simulink model "x4DOF_Model"  (R2023a)
settings: Solver=VariableStepAuto  StartTime=0.0  StopTime=60  RelTol=1e-3
InitFcn:
  | data = readtable("car_rig_data.xlsx");
settings Model: Creator=Sebastian  LastModifiedBy=Sebastian

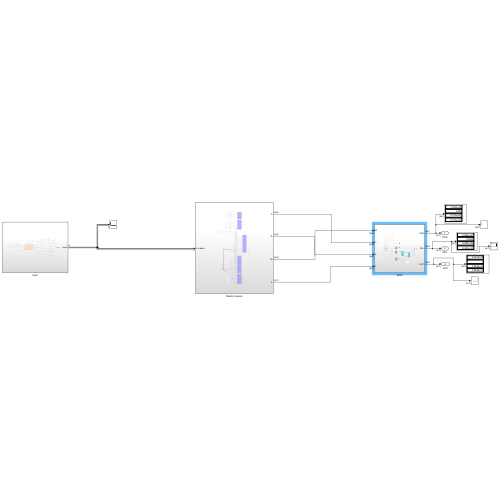
[thumbnail: Simulink's stored preview of the top-level diagram]
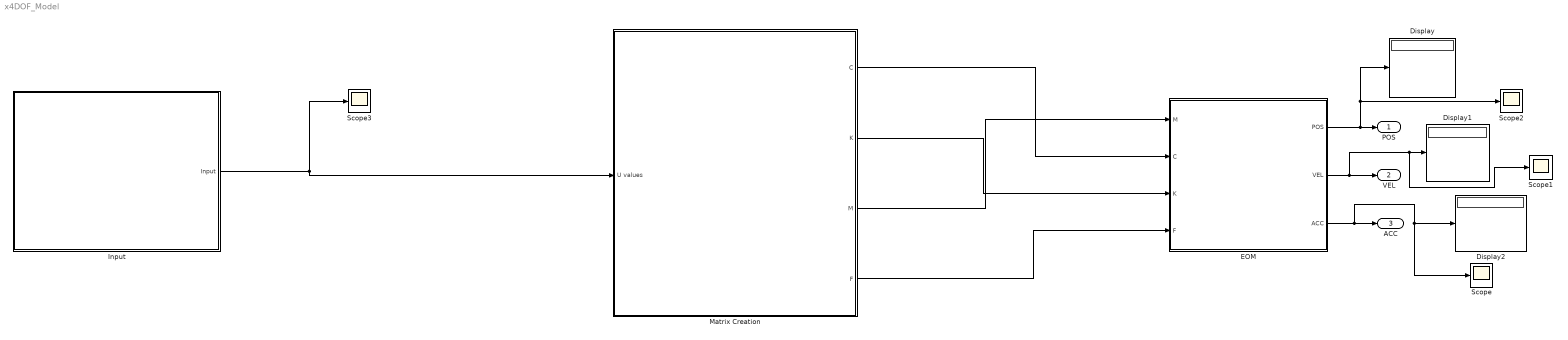
== system x4DOF_Model ==
  Display : Display
  Display1 : Display
  Display2 : Display
  EOM : Subsystem
  Input : Subsystem
  Matrix Creation : Subsystem
  Scope{,1..3} (4 alike) : Scope
  POS : Outport
  VEL : Outport  Port=2
  ACC : Outport  Port=3
  wires:
  Matrix Creation/3(M) -> EOM/1(M)
  Matrix Creation/2(K) -> EOM/3(K)
  Matrix Creation/1(C) -> EOM/2(C)
  Matrix Creation/4(F) -> EOM/4(F)
  EOM/1(POS) -> Scope2/1, Display/1, POS/1
  EOM/2(VEL) -> Scope1/1, Display1/1, VEL/1
  EOM/3(ACC) -> Scope/1, Display2/1, ACC/1
  Input/1(Input) -> Scope3/1, Matrix Creation/1(U values)

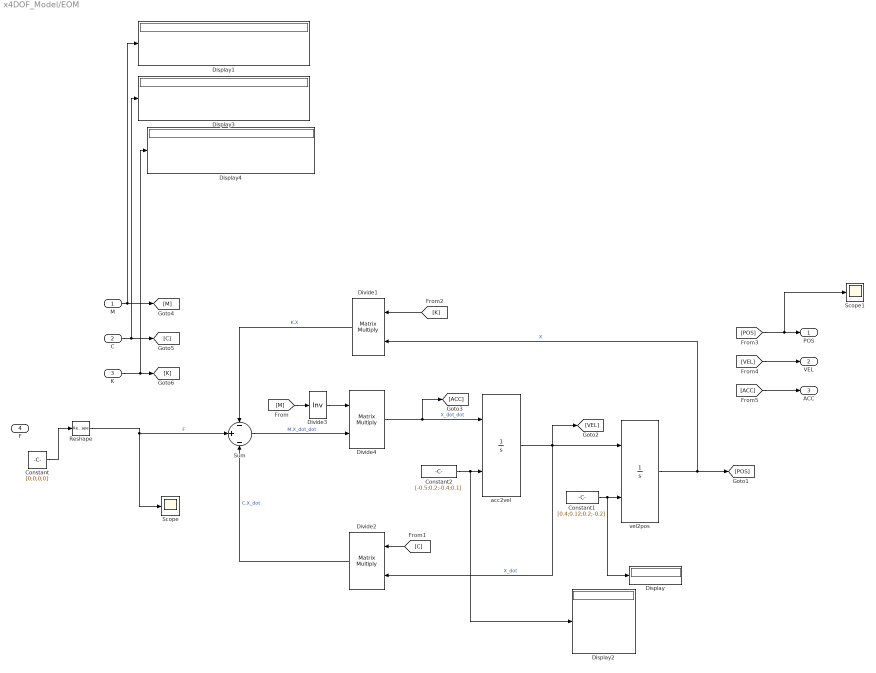
== system x4DOF_Model/EOM ==
  M : Inport
  C : Inport  Port=2
  K : Inport  Port=3
  F : Inport  Port=4
  Constant : Constant  Value=[0;0;0;0]
  Constant1 : Constant  Value=[0.4;0.12;0.2;-0.2]  VectorParams1D=off
  Constant2 : Constant  Value=[-0.5;0.2;-0.4;0.1]  VectorParams1D=off
  Display{,1..4} (5 alike) : Display
  Divide1 : Product  Multiplication=Matrix(*)
  Divide2 : Product  Multiplication=Matrix(*)
  Divide3 : Product  Inputs=/  Multiplication=Matrix(*)
  Divide4 : Product  Multiplication=Matrix(*)
  Reshape : Reshape  OutputDimensionality=Column vector (2-D)
  Scope : Scope
  Scope1 : Scope
  Sum : Sum  Inputs=-|+|-
  acc2vel : Integrator  InitialConditionSource=external
  vel2pos : Integrator  InitialConditionSource=external
  POS : Outport
  VEL : Outport  Port=2
  ACC : Outport  Port=3
  wires:
  Divide4/1 -> [ACC], acc2vel/1  "X_dot_dot"
  [C] -> Divide2/1
  vel2pos/1 -> [POS], Divide1/2  "X"
  Divide1/1 -> Sum/1  "K.X"
  acc2vel/1 -> vel2pos/1, [VEL], Divide2/2  "X_dot"
  [K] -> Divide1/1
  C/1 -> Display3/1, [C]
  Constant2/1 -> Display2/1, acc2vel/2
  [ACC] -> ACC/1
  [M] -> Divide3/1
  Constant1/1 -> Display/1, vel2pos/2
  [VEL] -> VEL/1
  Sum/1 -> Divide4/2  "M.X_dot_dot"
  Divide2/1 -> Sum/3  "C.X_dot"
  Divide3/1 -> Divide4/1
  Reshape/1 -> Scope/1, Sum/2  "F"
  [POS] -> Scope1/1, POS/1
  M/1 -> Display1/1, [M]
  K/1 -> Display4/1, [K]
  Constant/1 -> Reshape/1

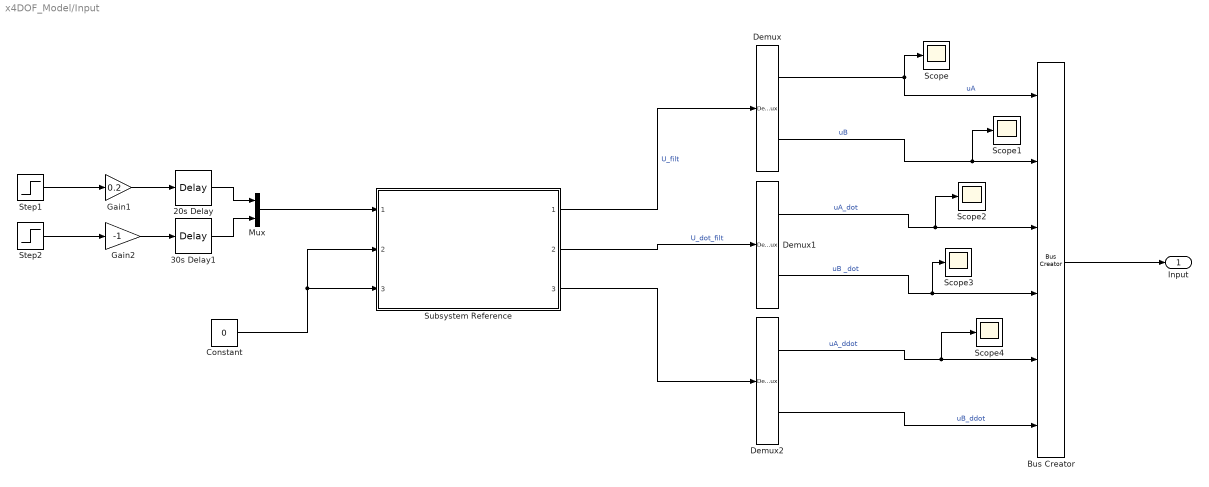
== system x4DOF_Model/Input ==
  20s Delay : TransportDelay  DelayTime=20
  30s Delay1 : TransportDelay  DelayTime=30
  Bus Creator : BusCreator  Inputs=6
  Constant : Constant  Value=0
  Demux : Demux  Outputs=2
  Demux1 : Demux  Outputs=2
  Demux2 : Demux  Outputs=2
  Gain1 : Gain  Gain=0.2
  Gain2 : Gain  Gain=-1
  Mux : Mux  Inputs=2
  Scope{,1..4} (5 alike) : Scope
  Step1 : Step  SampleTime=0
  Step2 : Step  SampleTime=0
  Subsystem Reference : Subsystem  ReferencedSubsystem=bh_COMPONENT_deriv_est  wn=2*pi*5000  p=1
  Input : Outport
  wires:
  Mux/1 -> Subsystem Reference/1
  Constant/1 -> Subsystem Reference/3, Subsystem Reference/2
  Subsystem Reference/1 -> Demux/1  "U_filt"
  Subsystem Reference/2 -> Demux1/1  "U_dot_filt"
  Subsystem Reference/3 -> Demux2/1
  Step2/1 -> Gain2/1
  Step1/1 -> Gain1/1
  Gain1/1 -> 20s Delay/1
  Gain2/1 -> 30s Delay1/1
  20s Delay/1 -> Mux/1
  30s Delay1/1 -> Mux/2
  Demux/1 -> Scope/1, Bus Creator/1  "uA"
  Demux/2 -> Bus Creator/2, Scope1/1  "uB"
  Demux1/1 -> Scope2/1, Bus Creator/3  "uA_dot"
  Demux1/2 -> Scope3/1, Bus Creator/4  "uB _dot"
  Demux2/1 -> Scope4/1, Bus Creator/5  "uA_ddot"
  Demux2/2 -> Bus Creator/6  "uB_ddot"
  Bus Creator/1 -> Input/1

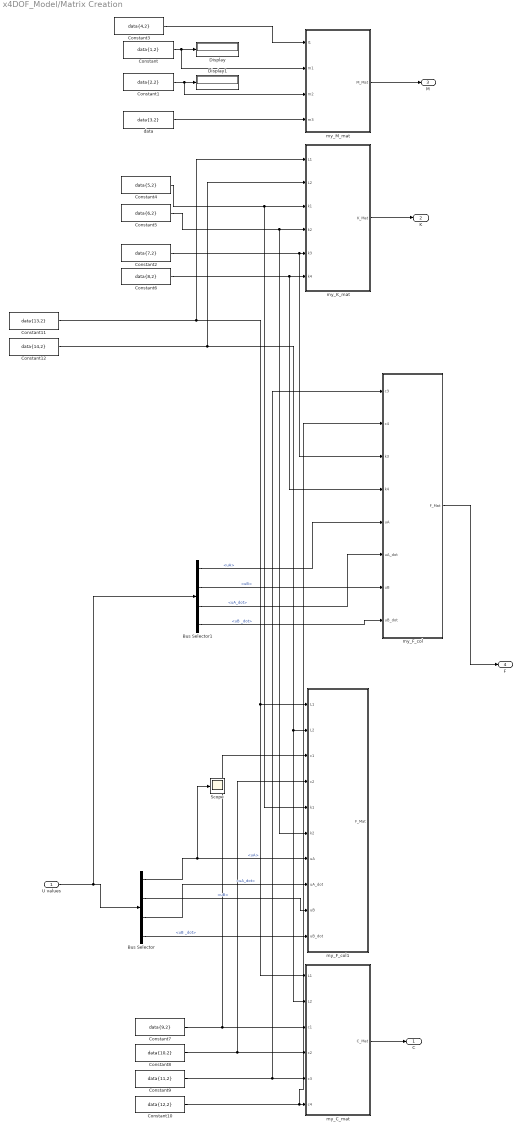
== system x4DOF_Model/Matrix Creation ==
  U values : Inport
  Bus Selector : BusSelector  OutputSignals=uA,uB,uA_dot,uB _dot
  Bus Selector1 : BusSelector  OutputSignals=uA,uB,uA_dot,uB _dot
  Constant : Constant  Value=data{1,2}
  Constant1 : Constant  Value=data{2,2}
  Constant10 : Constant  Value=data{12,2}
  Constant11 : Constant  Value=data{13,2}
  Constant12 : Constant  Value=data{14,2}
  Constant2 : Constant  Value=data{7,2}
  Constant3 : Constant  Value=data{4,2}
  Constant4 : Constant  Value=data{5,2}
  Constant5 : Constant  Value=data{6,2}
  Constant6 : Constant  Value=data{8,2}
  Constant7 : Constant  Value=data{9,2}
  Constant8 : Constant  Value=data{10,2}
  Constant9 : Constant  Value=data{11,2}
  Display : Display
  Display1 : Display
  Scope : Scope
  data : Constant  Value=data{3,2}
  my_C_mat : MATLAB Function  TreatAsAtomicUnit=on
  my_F_col : MATLAB Function  TreatAsAtomicUnit=on
  my_F_col1 : MATLAB Function  TreatAsAtomicUnit=on
  my_K_mat : MATLAB Function  TreatAsAtomicUnit=on
  my_M_mat : MATLAB Function  TreatAsAtomicUnit=on
  C : Outport
  K : Outport  Port=2
  M : Outport  Port=3
  F : Outport  Port=4
  wires:
  my_C_mat/1(C_Mat) -> C/1
  my_K_mat/1(K_Mat) -> K/1
  my_M_mat/1(M_Mat) -> M/1
  Constant/1 -> my_M_mat/2(m1), Display/1
  Constant1/1 -> my_M_mat/3(m2), Display1/1
  Constant3/1 -> my_M_mat/1(I1)
  data/1 -> my_M_mat/4(m3)
  Constant5/1 -> my_K_mat/4(k2), my_F_col1/6(k2)
  Constant4/1 -> my_F_col1/5(k1), my_K_mat/3(k1)
  Constant2/1 -> my_F_col/3(k3), my_K_mat/5(k3)
  Constant6/1 -> my_F_col/4(k4), my_K_mat/6(k4)
  Constant10/1 -> my_F_col/2(c4), my_C_mat/6(c4)
  Constant9/1 -> my_F_col/1(c3), my_C_mat/5(c3)
  Constant8/1 -> my_F_col1/4(c2), my_C_mat/4(c2)
  Constant7/1 -> my_C_mat/3(c1), my_F_col1/3(c1)
  Constant11/1 -> my_K_mat/1(L1), my_C_mat/1(L1), my_F_col1/1(L1)
  Constant12/1 -> my_K_mat/2(L2), my_C_mat/2(L2), my_F_col1/2(L2)
  Bus Selector/2 -> my_F_col1/9(uB)  "<uB>"
  U values/1 -> Bus Selector1/1, Bus Selector/1
  Bus Selector/4 -> my_F_col1/10(uB_dot)  "<uB _dot>"
  Bus Selector/3 -> my_F_col1/8(uA_dot)  "<uA_dot>"
  Bus Selector/1 -> Scope/1, my_F_col1/7(uA)  "<uA>"
  Bus Selector1/4 -> my_F_col/8(uB_dot)  "<uB _dot>"
  Bus Selector1/2 -> my_F_col/7(uB)  "<uB>"
  Bus Selector1/3 -> my_F_col/6(uA_dot)  "<uA_dot>"
  Bus Selector1/1 -> my_F_col/5(uA)  "<uA>"
  my_F_col/1(F_Mat) -> F/1

== matlab function x4DOF_Model/Matrix Creation/my_C_mat ==
  data: L1 input; C_Mat output; L2 input; c1 input; c2 input; c3 input; c4 input
function C_Mat = my_C_mat(L1,L2,c1,c2,c3,c4)
%#codegen

%    This function was generated by the Symbolic Math Toolbox version 9.3.
%    29-May-2023 20:31:21

% L1 = complex(L1);  % if required to enforce complex operations
% L2 = complex(L2);  % if required to enforce complex operations
% c1 = complex(c1);  % if required to enforce complex operations
% c2 = complex(c2);  % if required to enforce complex operations
% c3 = complex(c3);  % if required to enforce complex operations
% c4 = complex(c4);  % if required to enforce complex operations
t2 = L1.*c1;
t3 = L2.*c2;
t4 = -c1;
t5 = -c2;
C_Mat = reshape([t4+t5,-t2+t3,t4,t5,t2+t3,L1.*t2-L2.*t3,t2,t3,c1,t2,c1+c3,0.0,c2,-t3,0.0,c2+c4],[4,4]);
end

== matlab function x4DOF_Model/Matrix Creation/my_M_mat ==
  data: I1 input; M_Mat output; m1 input; m2 input; m3 input
function M_Mat = my_M_mat(I1,m1,m2,m3)
%#codegen

%    This function was generated by the Symbolic Math Toolbox version 9.3.
%    29-May-2023 20:31:20

% I1 = complex(I1);  % if required to enforce complex operations
% m1 = complex(m1);  % if required to enforce complex operations
% m2 = complex(m2);  % if required to enforce complex operations
% m3 = complex(m3);  % if required to enforce complex operations
M_Mat = reshape([m1,0.0,0.0,0.0,0.0,I1,0.0,0.0,0.0,0.0,m2,0.0,0.0,0.0,0.0,m3],[4,4]);
end

== matlab function x4DOF_Model/Matrix Creation/my_K_mat ==
  data: L1 input; K_Mat output; L2 input; k1 input; k2 input; k3 input; k4 input
function K_Mat = my_K_mat(L1,L2,k1,k2,k3,k4)
%#codegen

%    This function was generated by the Symbolic Math Toolbox version 9.3.
%    29-May-2023 20:31:21

% L1 = complex(L1);  % if required to enforce complex operations
% L2 = complex(L2);  % if required to enforce complex operations
% k1 = complex(k1);  % if required to enforce complex operations
% k2 = complex(k2);  % if required to enforce complex operations
% k3 = complex(k3);  % if required to enforce complex operations
% k4 = complex(k4);  % if required to enforce complex operations
t2 = L1.*k1;
t3 = L2.*k2;
t4 = -k1;
t5 = -k2;
K_Mat = reshape([t4+t5,-t2+t3,t4,t5,t2+t3,L1.*t2-L2.*t3,t2,t3,k1,t2,k1+k3,0.0,k2,-t3,0.0,k2+k4],[4,4]);
end

== matlab function x4DOF_Model/Matrix Creation/my_F_col ==
  data: c3 input; F_Mat output; c4 input; k3 input; k4 input; uA input; uA_dot input; uB input; uB_dot input
function F_Mat = my_F_col(c3,c4,k3,k4,uA,uA_dot,uB,uB_dot)
%#codegen

%    This function was generated by the Symbolic Math Toolbox version 9.3.
%    05-Jun-2023 14:32:45

% c3 = complex(c3);  % if required to enforce complex operations
% c4 = complex(c4);  % if required to enforce complex operations
% k3 = complex(k3);  % if required to enforce complex operations
% k4 = complex(k4);  % if required to enforce complex operations
% uA = complex(uA);  % if required to enforce complex operations
% uA_dot = complex(uA_dot);  % if required to enforce complex operations
% uB = complex(uB);  % if required to enforce complex operations
% uB_dot = complex(uB_dot);  % if required to enforce complex operations
F_Mat = [0.0;0.0;c3.*uA_dot+k3.*uA;c4.*uB_dot+k4.*uB];
end

== matlab function x4DOF_Model/Matrix Creation/my_F_col1 ==
  data: L1 input; F_Mat output; L2 input; c1 input; c2 input; k1 input; k2 input; uA input; uA_dot input; uB input; uB_dot input
function F_Mat = my_F_col(L1,L2,c1,c2,k1,k2,uA,uA_dot,uB,uB_dot)
%#codegen

%    This function was generated by the Symbolic Math Toolbox version 9.3.
%    05-Jun-2023 13:13:54

% L1 = complex(L1);  % if required to enforce complex operations
% L2 = complex(L2);  % if required to enforce complex operations
% c1 = complex(c1);  % if required to enforce complex operations
% c2 = complex(c2);  % if required to enforce complex operations
% k1 = complex(k1);  % if required to enforce complex operations
% k2 = complex(k2);  % if required to enforce complex operations
% uA = complex(uA);  % if required to enforce complex operations
% uA_dot = complex(uA_dot);  % if required to enforce complex operations
% uB = complex(uB);  % if required to enforce complex operations
% uB_dot = complex(uB_dot);  % if required to enforce complex operations
t2 = c1.*uA_dot;
t3 = c2.*uB_dot;
t4 = k1.*uA;
t5 = k2.*uB;
t6 = t2+t4;
t7 = t3+t5;
F_Mat = [t6+t7;L1.*t6-L2.*t7;t6;t7];
end
